simulink model "SCC"  (R2018a)
settings: Solver=ode23t  StartTime=0.0  StopTime=10.0  RelTol=1e-3
undefined symbols (not defined in the file): Ion, Lithium
libraries: powerlib x7, electricdrivelib x1, re_lib x1
settings Model: Creator=soura  LastModifiedBy=soura

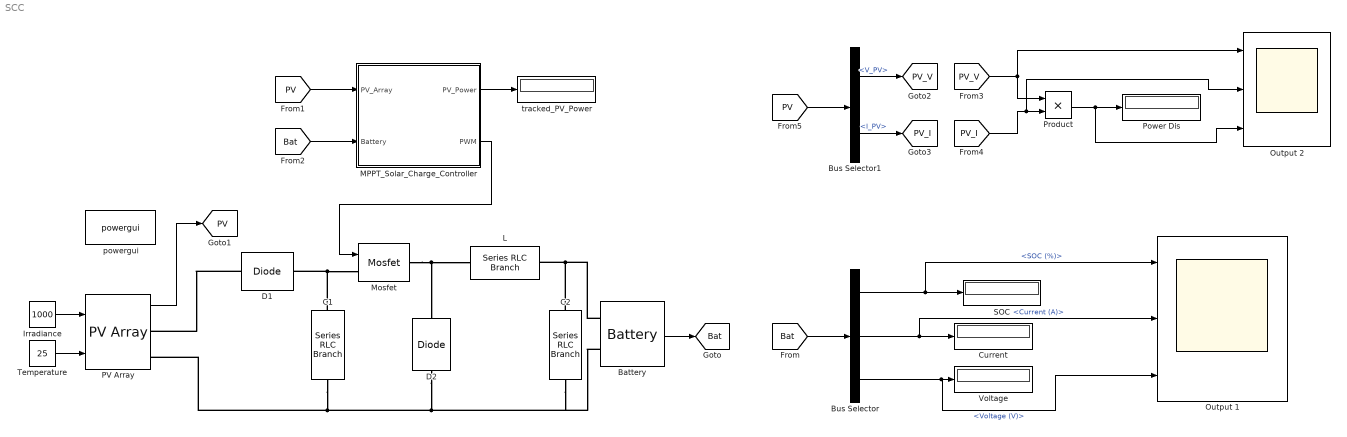
== system SCC ==
  Battery : electricdrivelib/Extra Sources/Battery  BatType=Lithium-Ion  ShowTempParam=off  ThermalPreset=no  ShowAgeParam=off  NomV=12  NomQ=5  SOC=20  Batt_Tr=1  PresetModel=on  MaxQ=5  MinV=9  FullV=13.9678  Dis_rate=2.1739  R=0.024  Normal_OP=4.5217  expZone="[12.9646     0.245652]"  current=[6.5 13 32.5]  Units=Time  Tci=20  NomT=20  T2=-30  MaxQ2=4.8  FullV2=7.1  Normal_OP2=5.655  expZone2="[6.58           1]"  Rca=0.6  ti=2000  Dp=0  Neq0=0  Tsim=1e6  Ta1=25  Qeol=5.4*0.9  Reol=0.013333*1.2  Char_age=[2.3478, 3]  Dis_age=[2.3478, 10]  N1=1500  N2=10500  N3=1000  N4=1400  Ta2=45  N5=950
  Bus Selector : BusSelector  OutputSignals=SOC (%),Current (A),Voltage (V)
  Bus Selector1 : BusSelector  OutputSignals=V_PV,I_PV
  C1 : powerlib/Elements/Series RLC Branch  LConnTagsString=__new0  RConnTagsString=__new0  BranchType=C  Resistance=1  Inductance=1e-3  SetiL0=off  InitialCurrent=0  Capacitance=1000e-6  Setx0=off  InitialVoltage=0  Measurements=None
  C2 : powerlib/Elements/Series RLC Branch  LConnTagsString=__new0  RConnTagsString=__new0  BranchType=C  Resistance=1  Inductance=1e-3  SetiL0=off  InitialCurrent=0  Capacitance=1000e-6  Setx0=off  InitialVoltage=0  Measurements=None
  Current : Display
  D1 : powerlib/Power Electronics/Diode  Ron=0.001  Lon=0  Vf=0.8  IC=0  UseSnubber=0  Rs=inf  Cs=0  Measurements=off
  D2 : powerlib/Power Electronics/Diode  Ron=0.001  Lon=0  Vf=0.5  IC=0  UseSnubber=0  Rs=inf  Cs=0  Measurements=off
  Irradiance : Constant  Value=1000
  L : powerlib/Elements/Series RLC Branch  LConnTagsString=__new0  RConnTagsString=__new0  BranchType=L  Resistance=1  Inductance=10e-3  SetiL0=off  InitialCurrent=0  Capacitance=1000e-6  Setx0=off  InitialVoltage=0  Measurements=None
  MPPT_Solar_Charge_Controller : Subsystem
  Mosfet : powerlib/Power Electronics/Mosfet  Ron=0.02  Lon=0  Rd=0.01  Vfd=0  IC=0  Rs=1e5  Cs=inf  Measurements=off
  Output 1 : Scope  NumInputPorts=3
  Output 2 : Scope  NumInputPorts=3
  PV Array : re_lib/Solar/PV Array  Npar=2  Nser=4  PlotType=array @ 25 deg.C & specified irradiances  S_vec="[ 1000  800 600 400 200 ]"  Temp_C_vec="[ 45 25  ]"  ModuleName=A10Green Technology A10J-S72-175  PlotWhenSelected=off  Pm=175.0914  Ncell=72  Voc=43.99  Isc=5.17  Vm=36.63  Im=4.78  beta_Voc_pc=-0.3616  alpha_Isc_pc=0.041509  beta_Voc=-0.15907  alpha_Isc=0.002146  IL=5.178  I0=1.7845e-10  nI=0.98852  Rsh=249.6783  Rs=0.38412  BAL=on  Tc=1e-6  Tfilter=5e-5
  Power Dis : Display
  Product : Product
  SOC : Display
  Temperature : Constant  Value=25
  Voltage : Display
  powergui : powerlib/powergui  Priority=1  SimulationMode=Discrete  SampleTime=1e-05  frequency=60  Iterations=50  frequencyindice=0  Pbase=100e6  ErrMax=1e-4  UnitsV=kV  UnitsW=MW  buscounter=0  FunctionMessages=off  echomessages=off  EnableUseOfTLC=off  CurrentSourceSwitches=off  DisableSnubberDevices=off  DisableRonSwitches=off  DisableVfSwitches=off  DisplayEquations=off  SolverType=Tustin/Backward Euler (TBE)  Interpol=off  ExternalGateDelay=off  methode=off  Ts=100  x0status=blocks  SPID=on  SwTol=0  HookPort=off  RestoreLinks=warning  ResistiveCurrentMeasurement=off  Frange=[0:2:500]  Ylog=off  Xlog=on  ShowGrid=off  save=off  variable=ZData  structure=0  ZoomFFT=off  StartTime=0.0  cycles=1  DisplayStyle=1  fundamental=60  FreqAxis=off  MaxFrequency=1000  frequencyindicesteady=1  RmsSteady=1  display=off
  tracked_PV_Power : Display
  tag scope: Bat=global, PV=global, PV_I=global, PV_V=global
  wires:
  Irradiance/1 -> PV Array/1
  Temperature/1 -> PV Array/2
  Bus Selector/1 -> Output 1/1, SOC/1  "<SOC (%)>"
  Bus Selector/2 -> Output 1/2, Current/1  "<Current (A)>"
  Bus Selector/3 -> Output 1/3, Voltage/1  "<Voltage (V)>"
  [Bat] -> Bus Selector/1
  Battery/1 -> [Bat]
  PV Array/1 -> [PV]
  [PV_I] -> Output 2/2, Product/2
  Product/1 -> Output 2/3, Power Dis/1
  [PV_V] -> Output 2/1, Product/1
  [PV] -> Bus Selector1/1
  Bus Selector1/1 -> [PV_V]  "<V_PV>"
  Bus Selector1/2 -> [PV_I]  "<I_PV>"
  [PV] -> MPPT_Solar_Charge_Controller/1(PV_Array)
  [Bat] -> MPPT_Solar_Charge_Controller/2(Battery)
  MPPT_Solar_Charge_Controller/1(PV_Power) -> tracked_PV_Power/1
  MPPT_Solar_Charge_Controller/2(PWM) -> Mosfet/1
  connections:
  D1/LConn1 -- PV Array/RConn1
  C1/LConn1 -- Mosfet/LConn1 -- D1/RConn1
  C1/RConn1 -- Battery/LConn2 -- C2/RConn1 -- D2/LConn1 -- PV Array/RConn2
  Mosfet/RConn1 -- L/RConn1 -- D2/RConn1
  C2/LConn1 -- Battery/LConn1 -- L/LConn1

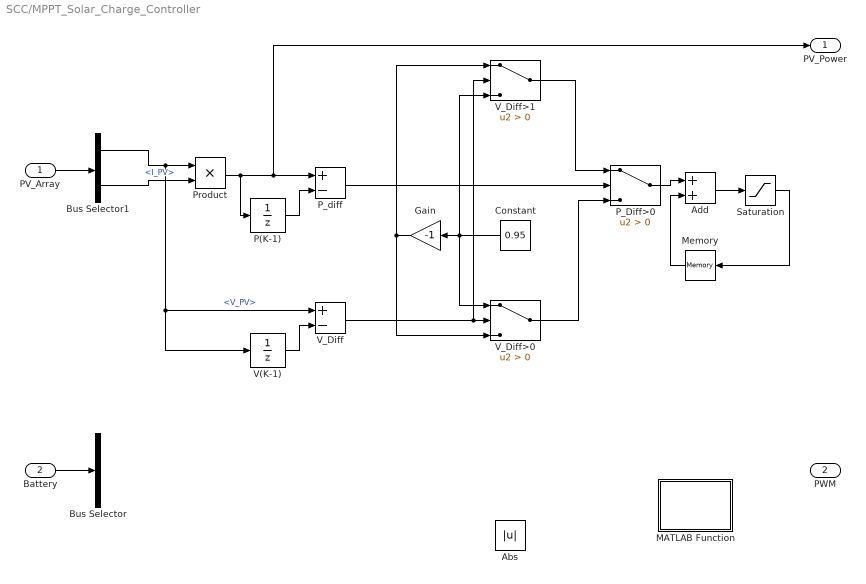
== system SCC/MPPT_Solar_Charge_Controller ==
  PV_Array : Inport
  Battery : Inport  Port=2
  Abs : Abs
  Add : Sum
  Bus Selector : BusSelector  OutputSignals=SOC (%),Current (A),Voltage (V)
  Bus Selector1 : BusSelector  OutputSignals=V_PV,I_PV
  Constant : Constant  Value=0.95  OutMin=[0]  OutMax=[0.95]
  Gain : Gain  Gain=-1
  MATLAB Function : MATLAB Function  TreatAsAtomicUnit=on
  Memory : Memory  InitialCondition=0.5  InheritSampleTime=on  LinearizeMemory=on  LinearizeAsDelay=on
  P(K-1) : UnitDelay  SampleTime=-1
  P_Diff>0 : Switch  Criteria=u2 > Threshold
  P_diff : Sum  Inputs=+-
  Product : Product
  Saturation : Saturate  UpperLimit=0.6  LowerLimit=0.4
  V(K-1) : UnitDelay  SampleTime=-1
  V_Diff : Sum  Inputs=+-
  V_Diff>0 : Switch  Criteria=u2 > Threshold
  V_Diff>1 : Switch  Criteria=u2 > Threshold
  PV_Power : Outport
  PWM : Outport  Port=2
  wires:
  PV_Array/1 -> Bus Selector1/1
  Bus Selector1/1 -> V(K-1)/1, V_Diff/1, Product/1  "<V_PV>"
  Bus Selector1/2 -> Product/2  "<I_PV>"
  Product/1 -> P(K-1)/1, PV_Power/1, P_diff/1
  P(K-1)/1 -> P_diff/2
  V(K-1)/1 -> V_Diff/2
  P_diff/1 -> P_Diff>0/2
  V_Diff/1 -> V_Diff>1/2, V_Diff>0/2
  V_Diff>0/1 -> P_Diff>0/3
  Gain/1 -> V_Diff>1/1, V_Diff>0/3
  V_Diff>1/1 -> P_Diff>0/1
  P_Diff>0/1 -> Add/1
  Memory/1 -> Add/2
  Add/1 -> Saturation/1
  Saturation/1 -> Memory/1
  Constant/1 -> V_Diff>1/3, V_Diff>0/1, Gain/1
  Battery/1 -> Bus Selector/1

== matlab function SCC/MPPT_Solar_Charge_Controller/MATLAB Function ==
function Duty_Cycle

end
